simulink model "punto6"  (R2019a)
settings: Solver=VariableStepAuto  StartTime=0.0  StopTime=10.0  MaxStep=1e-4  RelTol=1e-3
values from neighbouring files (symbols this model uses):
  alfa_cu = 3.9 * 10^(-3)    (= 0.0039)    [Datos.m]
  bl = 0    [Datos.m]
  bm = 1.5 * 10^(-5)    (= 1.5e-05)    [Datos.m]
  Cts = 0.818    [Datos.m]
  Id0 = 0.5    [Datos.m]    (also in punto6plot.m)
  Jl = 0.2520    (= 0.252)    [Datos.m]
  Jm = 3.1 * 10^(-6)    (= 3.1e-06)    [Datos.m]
  lambda_m_r = 0.01546    [Datos.m]
  Ld = 6.6e-3    (= 0.0066)    [Datos.m]
  Lq = 5.8e-3    (= 0.0058)    [Datos.m]
  Pp = 3    [Datos.m]
  r = 314.3008    [Datos.m]
  Rts_amb = 146.7    [Datos.m]
  Tlmax = 6.28    [Calculo.m]    (also in Datos.m)
  tstep1 = 0.1    [Calculo.m]    (also in Datos.m)
  tstep2 = 0.3    [Calculo.m]    (also in Datos.m)
  tstep4 = 0.7    [Calculo.m]    (also in Datos.m)
  tstep5 = 0.9    [Calculo.m]    (also in Datos.m)
  Vqsnom = 19.596    [Calculo.m]    (also in Datos.m)
undefined symbols (not defined in the file or in its folder): magnitude
settings Model: Creator=renzo  LastModifiedBy=renzo

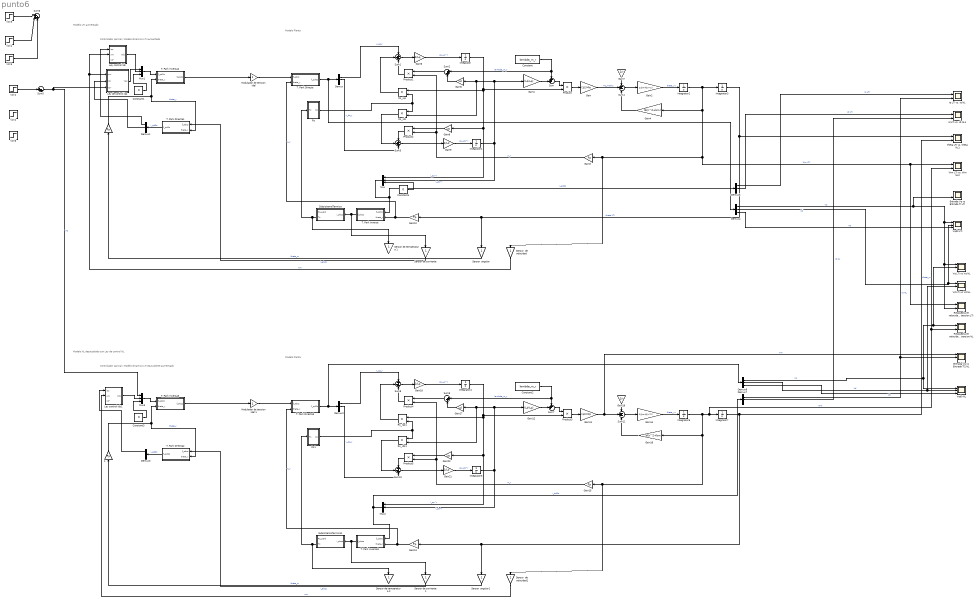
== system punto6 ==
  note: Modelo LTI aumentado
  note: Modelo Planta
  note: Controlador parcial / Modelo dinamico LTI aumentado
  note: Controlador parcial / Modelo dinamico LTI equivalente aumentado
  note: Modelo NL desacoplado con Ley de control NL
  note: Modelo Planta
  " " : Gain  Gain=Pp
  " 1" : Gain  Gain=Pp
  Constant : Constant  Value=lambda_m_r
  Constant1 : Constant  Value=0
  Constant2 : Constant  Value=lambda_m_r
  Constant3 : Constant  Value=0
  Constant4 : Constant  Value=0
  Demux{,1..5,7..8} (8 alike) : Demux  Outputs=3
  Entrada Vq vs Entrada Tl LTI : Scope  NumInputPorts=2
  Entrada Vq vs Entrada Tl2 NL : Scope  NumInputPorts=3
  Gain : Gain  Gain=(3/2)*Pp
  Gain1 : Gain  Gain=(Ld-Lq)
  Gain{3,10,13,15} (4 alike) : Gain  Gain=Pp
  Gain11 : Gain  Gain=(3/2)*Pp
  Gain12 : Gain  Gain=(Ld-Lq)
  Gain14 : Gain  Gain=1/(Jm+Jl/r^2)
  Gain16 : Gain  Gain=bl/r^2+bm
  Gain17 : Gain  Gain=Ld
  Gain18 : Gain  Gain=1/Lq
  Gain19 : Gain  Gain=1/r
  Gain2 : Gain  Gain=1/(Jm+Jl/r^2)
  Gain20 : Gain  Gain=Lq
  Gain21 : Gain  Gain=1/Ld
  Gain4 : Gain  Gain=(bl/r^2+bm)
  Gain5 : Gain  Gain=Ld
  Gain6 : Gain  Gain=1/Lq
  Gain7 : Gain  Gain=1/r
  Gain8 : Gain  Gain=Lq
  Gain9 : Gain  Gain=1/Ld
  Id LTI vs. Id NL1 : Scope  NumInputPorts=2
  Integrator{,2..4,6..7} (6 alike) : Integrator
  Integrator1 : Integrator  InitialCondition=Id0
  Integrator5 : Integrator  InitialCondition=Id0
  Iq LTI vs. Iq NL : Scope  NumInputPorts=2
  Ley control ids : Subsystem
  Ley control ids1 : Subsystem
  Ley de control iqs : Subsystem
  "Modulador de tension idel " : Gain
  Modulador de tension idel 1 : Gain
  Mux{,1..3} (4 alike) : Mux  Inputs=3
  Product{,1..5} (6 alike) : Product
  Respuesta en velocidad vs entrada tension LTI : Scope  NumInputPorts=2
  Respuesta en velocidad vs entrada tension NL : Scope  NumInputPorts=2
  Rs : Subsystem
  Rs1 : Subsystem
  Rs_ids : Product
  Rs_ids1 : Product
  Rs_iqs : Product
  Rs_iqs1 : Product
  Sensor  angular : Gain
  Sensor  angular1 : Gain
  Sensor  de velocidad : Gain
  Sensor  de velocidad1 : Gain
  "Sensor de corriente " : Gain
  Sensor de corriente 1 : Gain
  Sensor de temperatura 1 : Gain
  Sensor de temperatura 2 : Gain
  SubsistemaTermico : Subsystem
  SubsistemaTermico1 : Subsystem
  Sum : Sum  Inputs=++|
  Sum1 : Sum  Inputs=+--
  Sum10 : Sum  Inputs=+-+
  Sum11 : Sum  Inputs=-+-
  Sum2 : Sum  Inputs=|++
  Sum3 : Sum  Inputs=+-+
  Sum4 : Sum  Inputs=-+-
  Sum5 : Sum  Inputs=|++
  Sum6 : Sum  Inputs=|+++
  Sum7 : Sum  Inputs=++|
  Sum8 : Sum  Inputs=+--
  Sum9 : Sum  Inputs=|++
  T. Park Directa : Subsystem
  T. Park Directa1 : Subsystem
  T. Park Directa2 : Subsystem
  T. Park Directa3 : Subsystem
  T. Park Inversa : Subsystem
  T. Park Inversa2 : Subsystem
  T. Park Inversa3 : Subsystem
  T. Park Inversa5 : Subsystem
  V1*1 : Step  Time=tstep1  After=Vqsnom  SampleTime=0
  V1*2 : Step  Time=tstep4  After=-Vqsnom  SampleTime=0
  V1*3 : Step  Time=tstep2  After=Tlmax  SampleTime=0
  V1*4 : Step  Time=tstep4  After=-2*Tlmax  SampleTime=0
  V1*5 : Step  Time=tstep5  After=Tlmax  SampleTime=0
  V1*6 : Step  Time=0.5  After=0  SampleTime=0
  Vd LTI vs Vd NL : Scope  NumInputPorts=3
  Vq LTI vs Vq NL : Scope  NumInputPorts=3
  "Vqd0 LTI " : Scope  NumInputPorts=3
  "Vqd0 NL " : Scope  NumInputPorts=3
  Wm LTI vs. Wm NL2 : Scope  NumInputPorts=2
  theta LTI vs. theta NL1 : Scope  NumInputPorts=2
  wires:
  Gain8/1 -> Product2/1
  Sum1/1 -> Gain6/1
  Product2/1 -> Sum3/1
  Gain5/1 -> Sum2/2
  Demux/1 -> Sum1/1  "v_qs_r"
  Constant/1 -> Sum/1, Sum2/1  "lambda_m_r"
  Gain6/1 -> Integrator/1  "d_i_qr^r"
  Rs_iqs/1 -> Sum1/2
  Product1/1 -> Sum1/3
  Gain9/1 -> Integrator1/1  "d_i_ds^r"
  Integrator/1 -> Product/2, Mux/1, Gain8/1, Rs_iqs/1  "i_qs^r"
  Demux/2 -> Sum3/3  "v_ds_r"
  Gain1/1 -> Sum/2
  Sum2/1 -> Product1/1
  Sum3/1 -> Gain9/1
  Gain3/1 -> Product1/2, Product2/2  "w_r"
  Sum/1 -> Product/1
  Rs_ids/1 -> Sum3/2
  Integrator1/1 -> Gain5/1, Rs_ids/2, Gain1/1, Mux/2  "i_ds^r"
  Mux/1 -> T. Park Inversa/1(f_qd0s), Demux5/1  "i_qd0s"
  Product/1 -> Gain/1
  Gain2/1 -> Integrator2/1  "theta_vv"
  Gain4/1 -> Sum4/3
  Gain/1 -> Sum4/2  "Tq_motriz"
  Sum4/1 -> Gain2/1
  Rs/1(Rs) -> Rs_ids/1, Rs_iqs/2
  SubsistemaTermico/2(Ts) -> Sensor de temperatura 1/1, Rs/1(Ts)
  Gain7/1 -> Sum4/1
  T. Park Inversa/1(f_abcs) -> "Sensor de corriente "/1, SubsistemaTermico/1(i_abcs)
  " "/1 -> T. Park Inversa2/2(theta_r), T. Park Directa1/2(theta_r)  "theta_r"
  T. Park Directa1/1(f_qd0s) -> Demux1/1  "i_qd0s"
  Constant1/1 -> Mux1/3
  Ley control ids/1(Vds) -> Mux1/2
  Ley de control iqs/1(Vqs) -> Mux1/1
  Demux1/2 -> Ley de control iqs/2(ids)
  Demux1/1 -> Ley control ids/1(iqs)
  Mux1/1 -> T. Park Inversa2/1(f_qd0s)
  Gain10/1 -> T. Park Directa/2(theta_r), T. Park Inversa/2(theta_r)  "w_r"
  "Modulador de tension idel "/1 -> T. Park Directa/1(f_abcs)
  T. Park Inversa2/1(f_abcs) -> "Modulador de tension idel "/1
  "Sensor de corriente "/1 -> T. Park Directa1/1(f_abcs)  "i_abcs"
  Sensor  angular/1 -> " "/1  "theta_m"
  Sensor  de velocidad/1 -> Ley control ids/2(wm), Ley de control iqs/1(wm)  "wm"
  V1*1/1 -> Sum5/1
  V1*3/1 -> Sum6/1
  V1*5/1 -> Sum6/3
  V1*4/1 -> Sum6/2
  Sum5/1 -> Mux3/1, Ley de control iqs/3(Vq*)  "Vq"
  Mux3/1 -> T. Park Inversa5/1(f_qd0s)
  Ley control ids1/1(Vds) -> Mux3/2
  Constant3/1 -> Mux3/3
  T. Park Directa2/1(f_qd0s) -> Demux3/1  "i_qd0s"
  " 1"/1 -> T. Park Inversa5/2(theta_r), T. Park Directa2/2(theta_r)  "theta_r"
  Sensor  angular1/1 -> " 1"/1  "theta_m"
  T. Park Inversa3/1(f_abcs) -> Sensor de corriente 1/1, SubsistemaTermico1/1(i_abcs)
  Gain14/1 -> Integrator6/1  "theta_vv"
  Rs1/1(Rs) -> Rs_ids1/1, Rs_iqs1/2
  Product3/1 -> Gain11/1
  Rs_ids1/1 -> Sum10/2
  Gain15/1 -> Product4/2, Product5/2  "w_r"
  Sum7/1 -> Product3/1
  Gain16/1 -> Sum11/3
  Gain19/1 -> Sum11/1
  Sum10/1 -> Gain21/1
  Sum9/1 -> Product4/1
  Demux2/2 -> Sum10/3  "v_ds_r"
  Gain21/1 -> Integrator5/1  "d_i_ds^r"
  Rs_iqs1/1 -> Sum8/2
  Product4/1 -> Sum8/3
  Gain18/1 -> Integrator4/1  "d_i_qr^r"
  Constant2/1 -> Sum7/1, Sum9/1  "lambda_m_r"
  Sum8/1 -> Gain18/1
  Product5/1 -> Sum10/1
  Gain17/1 -> Sum9/2
  Integrator4/1 -> Product3/2, Mux2/1, Gain20/1, Rs_iqs1/1  "i_qs^r"
  Gain20/1 -> Product5/1
  Demux2/1 -> Sum8/1  "v_qs_r"
  Modulador de tension idel 1/1 -> T. Park Directa3/1(f_abcs)
  Sum11/1 -> Gain14/1
  SubsistemaTermico1/2(Ts) -> Sensor de temperatura 2/1, Rs1/1(Ts)
  T. Park Directa3/1(f_qd0s) -> Demux8/1, Demux2/1
  Sensor de corriente 1/1 -> T. Park Directa2/1(f_abcs)  "i_abcs"
  Mux2/1 -> T. Park Inversa3/1(f_qd0s), Demux7/1  "i_qd0s"
  Gain12/1 -> Sum7/2
  Gain13/1 -> T. Park Directa3/2(theta_r), T. Park Inversa3/2(theta_r)  "w_r"
  Sensor  de velocidad1/1 -> Ley control ids1/2(wm)  "wm"
  Integrator5/1 -> Gain17/1, Rs_ids1/2, Gain12/1, Mux2/2  "i_ds^r"
  T. Park Inversa5/1(f_abcs) -> Modulador de tension idel 1/1
  Demux7/1 -> Iq LTI vs. Iq NL/2, Entrada Vq vs Entrada Tl2 NL/2  "Iq NL"
  Gain11/1 -> Entrada Vq vs Entrada Tl2 NL/1, Sum11/2  "Tm"
  Demux5/2 -> Id LTI vs. Id NL1/1  "Id LTI"
  Integrator3/1 -> theta LTI vs. theta NL1/1, Sensor  angular/1, Gain10/1  "theta LTI"
  Integrator6/1 -> Sensor  de velocidad1/1, Gain15/1, Gain16/1, Respuesta en velocidad vs entrada tension NL/2, Wm LTI vs. Wm NL2/2, Integrator7/1  "Wm"
  Demux7/2 -> Id LTI vs. Id NL1/2  "Id NL"
  Integrator2/1 -> Respuesta en velocidad vs entrada tension LTI/1, Wm LTI vs. Wm NL2/1, Sensor  de velocidad/1, Gain3/1, Gain4/1, Integrator3/1  "Wm LTI"
  Demux4/2 -> "Vqd0 LTI "/2, Vd LTI vs Vd NL/1  "Vd"
  Integrator7/1 -> theta LTI vs. theta NL1/2, Sensor  angular1/1, Gain13/1  "theta_m"
  Demux4/1 -> Respuesta en velocidad vs entrada tension LTI/2, Vq LTI vs Vq NL/1, "Vqd0 LTI "/1, Entrada Vq vs Entrada Tl LTI/2  "Vq"
  Demux4/3 -> "Vqd0 LTI "/3  "V0"
  Demux5/1 -> Iq LTI vs. Iq NL/1  "Iq LTI"
  T. Park Directa/1(f_qd0s) -> Demux4/1, Demux/1
  Demux8/1 -> Respuesta en velocidad vs entrada tension NL/1, Vq LTI vs Vq NL/2, "Vqd0 NL "/1  "Vq"
  Demux8/2 -> "Vqd0 NL "/2, Vd LTI vs Vd NL/2  "Vd"
  Demux8/3 -> "Vqd0 NL "/3  "V0"
  Demux3/1 -> Ley control ids1/1(iqs)
  Constant4/1 -> Mux/3

== system punto6/Ley control ids ==
  iqs : Inport
  wm : Inport  Port=2
  Vd* : Inport  Port=3
  Ley de Control minima : Subsystem
  Sum : Sum  Inputs=|-+
  Vds : Outport
  wires:
  wm/1 -> Ley de Control minima/2(wm)
  iqs/1 -> Ley de Control minima/1(Iqs)
  Ley de Control minima/1(Vds*) -> Sum/1
  Sum/1 -> Vds/1
  Vd*/1 -> Sum/2

== system punto6/Ley control ids1 ==
  iqs : Inport
  wm : Inport  Port=2
  Vd* : Inport  Port=3
  Ley de Control minima : Subsystem
  Sum : Sum  Inputs=|-+
  Vds : Outport
  wires:
  wm/1 -> Ley de Control minima/2(wm)
  iqs/1 -> Ley de Control minima/1(Iqs)
  Ley de Control minima/1(Vds*) -> Sum/1
  Sum/1 -> Vds/1
  Vd*/1 -> Sum/2

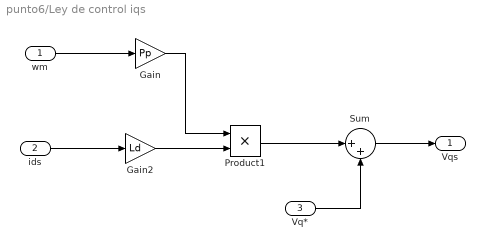
== system punto6/Ley de control iqs ==
  wm : Inport
  ids : Inport  Port=2
  Vq* : Inport  Port=3
  Gain : Gain  Gain=Pp
  Gain2 : Gain  Gain=Ld
  Product1 : Product
  Sum : Sum  Inputs=|++
  Vqs : Outport
  wires:
  wm/1 -> Gain/1
  Gain/1 -> Product1/1
  ids/1 -> Gain2/1
  Gain2/1 -> Product1/2
  Product1/1 -> Sum/1
  Sum/1 -> Vqs/1
  Vq*/1 -> Sum/2

== system punto6/Rs ==
  Ts : Inport
  Rs_ref : Gain  Gain=1.02
  Sum5 : Sum  Inputs=|+-
  Sum6 : Sum  Inputs=|++
  Ts_ref : Constant  Value=40
  alfa_cu : Gain  Gain=alfa_cu
  cte : Constant
  Rs : Outport
  wires:
  Ts_ref/1 -> Sum5/2
  Sum5/1 -> alfa_cu/1
  Sum6/1 -> Rs_ref/1
  Ts/1 -> Sum5/1
  alfa_cu/1 -> Sum6/1
  cte/1 -> Sum6/2
  Rs_ref/1 -> Rs/1  "Rs"

== system punto6/Rs1 ==
  Ts : Inport
  Rs_ref : Gain  Gain=1.02
  Sum5 : Sum  Inputs=|+-
  Sum6 : Sum  Inputs=|++
  Ts_ref : Constant  Value=40
  alfa_cu : Gain  Gain=alfa_cu
  cte : Constant
  Rs : Outport
  wires:
  Ts_ref/1 -> Sum5/2
  Sum5/1 -> alfa_cu/1
  Sum6/1 -> Rs_ref/1
  Ts/1 -> Sum5/1
  alfa_cu/1 -> Sum6/1
  cte/1 -> Sum6/2
  Rs_ref/1 -> Rs/1  "Rs"

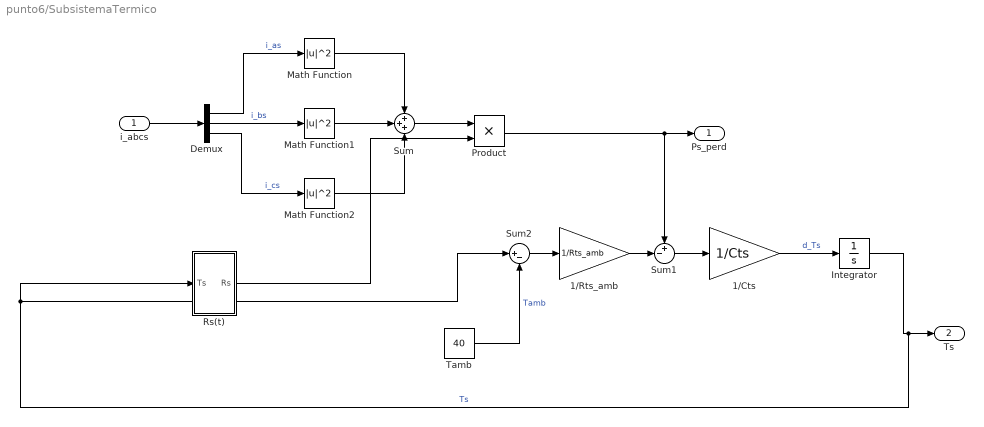
== system punto6/SubsistemaTermico ==
  i_abcs : Inport
  1/Cts : Gain  Gain=1/Cts
  1/Rts_amb : Gain  Gain=1/Rts_amb
  Demux : Demux  Outputs=3
  Integrator : Integrator  InitialCondition=40
  Math Function : Math  Operator=magnitude^2  SaturateOnIntegerOverflow=on
  Math Function1 : Math  Operator=magnitude^2  SaturateOnIntegerOverflow=on
  Math Function2 : Math  Operator=magnitude^2  SaturateOnIntegerOverflow=on
  Product : Product
  Rs(t) : Subsystem
  Sum : Sum  Inputs=3
  Sum1 : Sum  Inputs=+-|
  Sum2 : Sum  Inputs=|+-
  Tamb : Constant  Value=40
  Ps_perd : Outport  VectorParamsAs1DForOutWhenUnconnected=on
  Ts : Outport  Port=2  VectorParamsAs1DForOutWhenUnconnected=on
  wires:
  i_abcs/1 -> Demux/1
  Demux/1 -> Math Function/1  "i_as"
  Demux/2 -> Math Function1/1  "i_bs"
  Demux/3 -> Math Function2/1  "i_cs"
  Math Function1/1 -> Sum/2
  Math Function/1 -> Sum/1
  Math Function2/1 -> Sum/3
  Sum/1 -> Product/1
  Product/1 -> Sum1/1, Ps_perd/1
  Tamb/1 -> Sum2/2  "Tamb"
  Sum2/1 -> 1/Rts_amb/1
  1/Rts_amb/1 -> Sum1/2
  Sum1/1 -> 1/Cts/1
  1/Cts/1 -> Integrator/1  "d_Ts"
  Integrator/1 -> Rs(t)/1(Ts), Sum2/1, Ts/1  "Ts"
  Rs(t)/1(Rs) -> Product/2

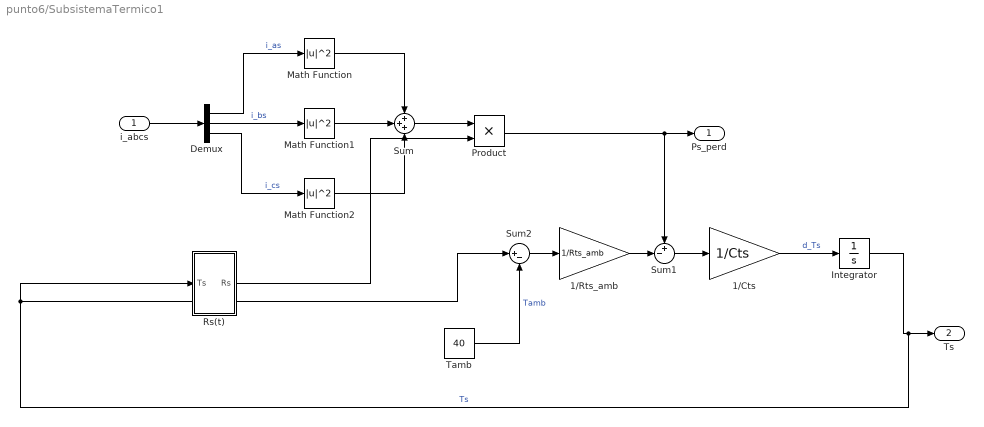
== system punto6/SubsistemaTermico1 ==
  i_abcs : Inport
  1/Cts : Gain  Gain=1/Cts
  1/Rts_amb : Gain  Gain=1/Rts_amb
  Demux : Demux  Outputs=3
  Integrator : Integrator  InitialCondition=40
  Math Function : Math  Operator=magnitude^2  SaturateOnIntegerOverflow=on
  Math Function1 : Math  Operator=magnitude^2  SaturateOnIntegerOverflow=on
  Math Function2 : Math  Operator=magnitude^2  SaturateOnIntegerOverflow=on
  Product : Product
  Rs(t) : Subsystem
  Sum : Sum  Inputs=3
  Sum1 : Sum  Inputs=+-|
  Sum2 : Sum  Inputs=|+-
  Tamb : Constant  Value=40
  Ps_perd : Outport  VectorParamsAs1DForOutWhenUnconnected=on
  Ts : Outport  Port=2  VectorParamsAs1DForOutWhenUnconnected=on
  wires:
  i_abcs/1 -> Demux/1
  Demux/1 -> Math Function/1  "i_as"
  Demux/2 -> Math Function1/1  "i_bs"
  Demux/3 -> Math Function2/1  "i_cs"
  Math Function1/1 -> Sum/2
  Math Function/1 -> Sum/1
  Math Function2/1 -> Sum/3
  Sum/1 -> Product/1
  Product/1 -> Sum1/1, Ps_perd/1
  Tamb/1 -> Sum2/2  "Tamb"
  Sum2/1 -> 1/Rts_amb/1
  1/Rts_amb/1 -> Sum1/2
  Sum1/1 -> 1/Cts/1
  1/Cts/1 -> Integrator/1  "d_Ts"
  Integrator/1 -> Rs(t)/1(Ts), Sum2/1, Ts/1  "Ts"
  Rs(t)/1(Rs) -> Product/2

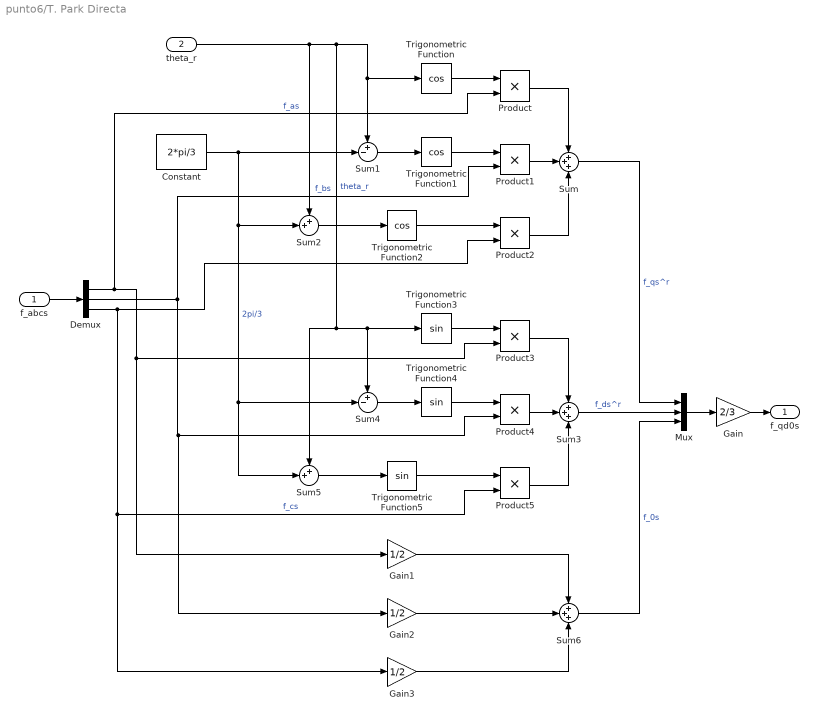
== system punto6/T. Park Directa ==
  f_abcs : Inport
  theta_r : Inport  Port=2
  Constant : Constant  Value=2*pi/3
  Demux : Demux  Outputs=3
  Gain : Gain  Gain=2/3
  Gain1 : Gain  Gain=1/2
  Gain2 : Gain  Gain=1/2
  Gain3 : Gain  Gain=1/2
  Mux : Mux  Inputs=3
  Product{,1..5} (6 alike) : Product
  Sum : Sum  Inputs=3
  Sum1 : Sum  Inputs=+-|
  Sum2 : Sum  Inputs=++|
  Sum3 : Sum  Inputs=3
  Sum4 : Sum  Inputs=+-|
  Sum5 : Sum  Inputs=++|
  Sum6 : Sum  Inputs=3
  Trigonometric Function : Trigonometry  Operator=cos
  Trigonometric Function1 : Trigonometry  Operator=cos
  Trigonometric Function2 : Trigonometry  Operator=cos
  Trigonometric Function3 : Trigonometry
  Trigonometric Function4 : Trigonometry
  Trigonometric Function5 : Trigonometry
  f_qd0s : Outport  VectorParamsAs1DForOutWhenUnconnected=on
  wires:
  Mux/1 -> Gain/1
  f_abcs/1 -> Demux/1
  Demux/1 -> Gain1/1, Product3/2, Product/2  "f_as"
  Demux/2 -> Gain2/1, Product4/2, Product1/2  "f_bs"
  Demux/3 -> Gain3/1, Product5/2, Product2/2  "f_cs"
  Sum/1 -> Mux/1  "f_qs^r"
  Gain/1 -> f_qd0s/1
  Trigonometric Function/1 -> Product/1
  Product/1 -> Sum/1
  Sum1/1 -> Trigonometric Function1/1
  Constant/1 -> Sum5/2, Sum4/2, Sum2/2, Sum1/2  "2pi/3"
  Trigonometric Function1/1 -> Product1/1
  Product1/1 -> Sum/2
  Product2/1 -> Sum/3
  Trigonometric Function2/1 -> Product2/1
  Sum2/1 -> Trigonometric Function2/1
  Product4/1 -> Sum3/2
  Trigonometric Function5/1 -> Product5/1
  Sum5/1 -> Trigonometric Function5/1
  Product5/1 -> Sum3/3
  Product3/1 -> Sum3/1
  Trigonometric Function4/1 -> Product4/1
  Sum4/1 -> Trigonometric Function4/1
  Sum3/1 -> Mux/2  "f_ds^r"
  Trigonometric Function3/1 -> Product3/1
  theta_r/1 -> Sum5/1, Sum4/1, Trigonometric Function3/1, Trigonometric Function/1, Sum1/1, Sum2/1  "theta_r"
  Sum6/1 -> Mux/3  "f_0s"
  Gain3/1 -> Sum6/3
  Gain1/1 -> Sum6/1
  Gain2/1 -> Sum6/2

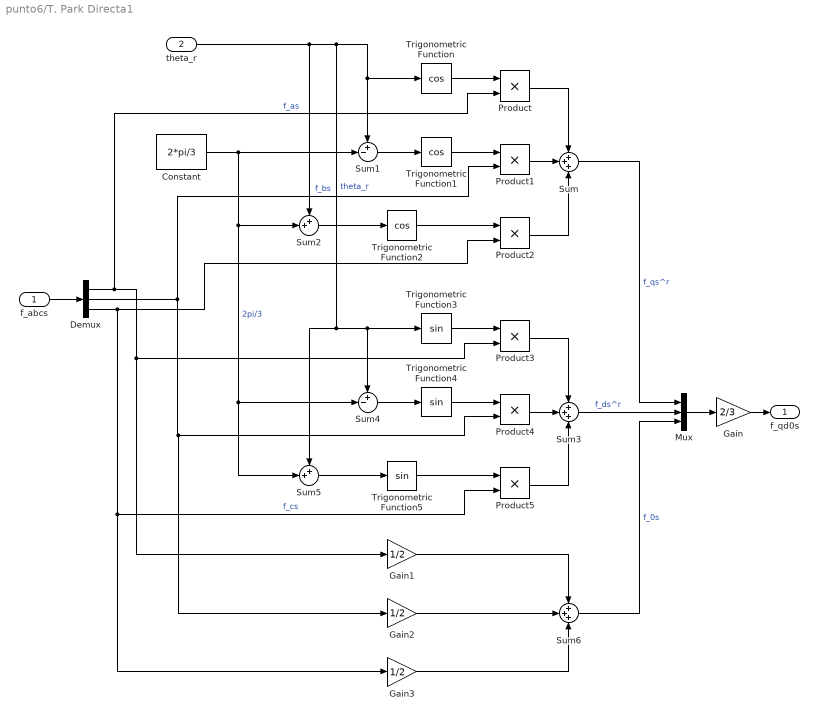
== system punto6/T. Park Directa1 ==
  f_abcs : Inport
  theta_r : Inport  Port=2
  Constant : Constant  Value=2*pi/3
  Demux : Demux  Outputs=3
  Gain : Gain  Gain=2/3
  Gain1 : Gain  Gain=1/2
  Gain2 : Gain  Gain=1/2
  Gain3 : Gain  Gain=1/2
  Mux : Mux  Inputs=3
  Product{,1..5} (6 alike) : Product
  Sum : Sum  Inputs=3
  Sum1 : Sum  Inputs=+-|
  Sum2 : Sum  Inputs=++|
  Sum3 : Sum  Inputs=3
  Sum4 : Sum  Inputs=+-|
  Sum5 : Sum  Inputs=++|
  Sum6 : Sum  Inputs=3
  Trigonometric Function : Trigonometry  Operator=cos
  Trigonometric Function1 : Trigonometry  Operator=cos
  Trigonometric Function2 : Trigonometry  Operator=cos
  Trigonometric Function3 : Trigonometry
  Trigonometric Function4 : Trigonometry
  Trigonometric Function5 : Trigonometry
  f_qd0s : Outport  VectorParamsAs1DForOutWhenUnconnected=on
  wires:
  Mux/1 -> Gain/1
  f_abcs/1 -> Demux/1
  Demux/1 -> Gain1/1, Product3/2, Product/2  "f_as"
  Demux/2 -> Gain2/1, Product4/2, Product1/2  "f_bs"
  Demux/3 -> Gain3/1, Product5/2, Product2/2  "f_cs"
  Sum/1 -> Mux/1  "f_qs^r"
  Gain/1 -> f_qd0s/1
  Trigonometric Function/1 -> Product/1
  Product/1 -> Sum/1
  Sum1/1 -> Trigonometric Function1/1
  Constant/1 -> Sum5/2, Sum4/2, Sum2/2, Sum1/2  "2pi/3"
  Trigonometric Function1/1 -> Product1/1
  Product1/1 -> Sum/2
  Product2/1 -> Sum/3
  Trigonometric Function2/1 -> Product2/1
  Sum2/1 -> Trigonometric Function2/1
  Product4/1 -> Sum3/2
  Trigonometric Function5/1 -> Product5/1
  Sum5/1 -> Trigonometric Function5/1
  Product5/1 -> Sum3/3
  Product3/1 -> Sum3/1
  Trigonometric Function4/1 -> Product4/1
  Sum4/1 -> Trigonometric Function4/1
  Sum3/1 -> Mux/2  "f_ds^r"
  Trigonometric Function3/1 -> Product3/1
  theta_r/1 -> Sum5/1, Sum4/1, Trigonometric Function3/1, Trigonometric Function/1, Sum1/1, Sum2/1  "theta_r"
  Sum6/1 -> Mux/3  "f_0s"
  Gain3/1 -> Sum6/3
  Gain1/1 -> Sum6/1
  Gain2/1 -> Sum6/2

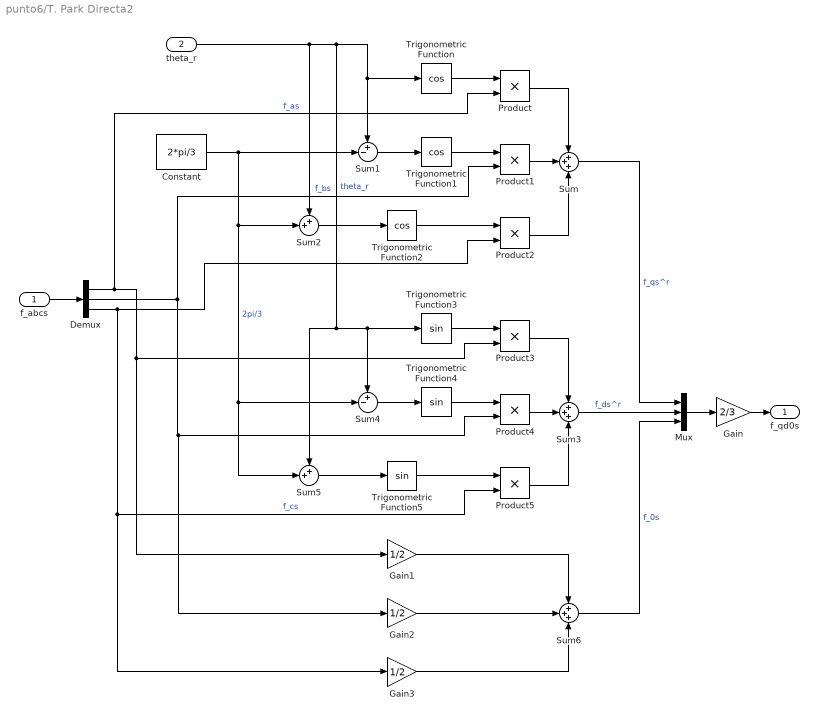
== system punto6/T. Park Directa2 ==
  f_abcs : Inport
  theta_r : Inport  Port=2
  Constant : Constant  Value=2*pi/3
  Demux : Demux  Outputs=3
  Gain : Gain  Gain=2/3
  Gain1 : Gain  Gain=1/2
  Gain2 : Gain  Gain=1/2
  Gain3 : Gain  Gain=1/2
  Mux : Mux  Inputs=3
  Product{,1..5} (6 alike) : Product
  Sum : Sum  Inputs=3
  Sum1 : Sum  Inputs=+-|
  Sum2 : Sum  Inputs=++|
  Sum3 : Sum  Inputs=3
  Sum4 : Sum  Inputs=+-|
  Sum5 : Sum  Inputs=++|
  Sum6 : Sum  Inputs=3
  Trigonometric Function : Trigonometry  Operator=cos
  Trigonometric Function1 : Trigonometry  Operator=cos
  Trigonometric Function2 : Trigonometry  Operator=cos
  Trigonometric Function3 : Trigonometry
  Trigonometric Function4 : Trigonometry
  Trigonometric Function5 : Trigonometry
  f_qd0s : Outport  VectorParamsAs1DForOutWhenUnconnected=on
  wires:
  Mux/1 -> Gain/1
  f_abcs/1 -> Demux/1
  Demux/1 -> Gain1/1, Product3/2, Product/2  "f_as"
  Demux/2 -> Gain2/1, Product4/2, Product1/2  "f_bs"
  Demux/3 -> Gain3/1, Product5/2, Product2/2  "f_cs"
  Sum/1 -> Mux/1  "f_qs^r"
  Gain/1 -> f_qd0s/1
  Trigonometric Function/1 -> Product/1
  Product/1 -> Sum/1
  Sum1/1 -> Trigonometric Function1/1
  Constant/1 -> Sum5/2, Sum4/2, Sum2/2, Sum1/2  "2pi/3"
  Trigonometric Function1/1 -> Product1/1
  Product1/1 -> Sum/2
  Product2/1 -> Sum/3
  Trigonometric Function2/1 -> Product2/1
  Sum2/1 -> Trigonometric Function2/1
  Product4/1 -> Sum3/2
  Trigonometric Function5/1 -> Product5/1
  Sum5/1 -> Trigonometric Function5/1
  Product5/1 -> Sum3/3
  Product3/1 -> Sum3/1
  Trigonometric Function4/1 -> Product4/1
  Sum4/1 -> Trigonometric Function4/1
  Sum3/1 -> Mux/2  "f_ds^r"
  Trigonometric Function3/1 -> Product3/1
  theta_r/1 -> Sum5/1, Sum4/1, Trigonometric Function3/1, Trigonometric Function/1, Sum1/1, Sum2/1  "theta_r"
  Sum6/1 -> Mux/3  "f_0s"
  Gain3/1 -> Sum6/3
  Gain1/1 -> Sum6/1
  Gain2/1 -> Sum6/2

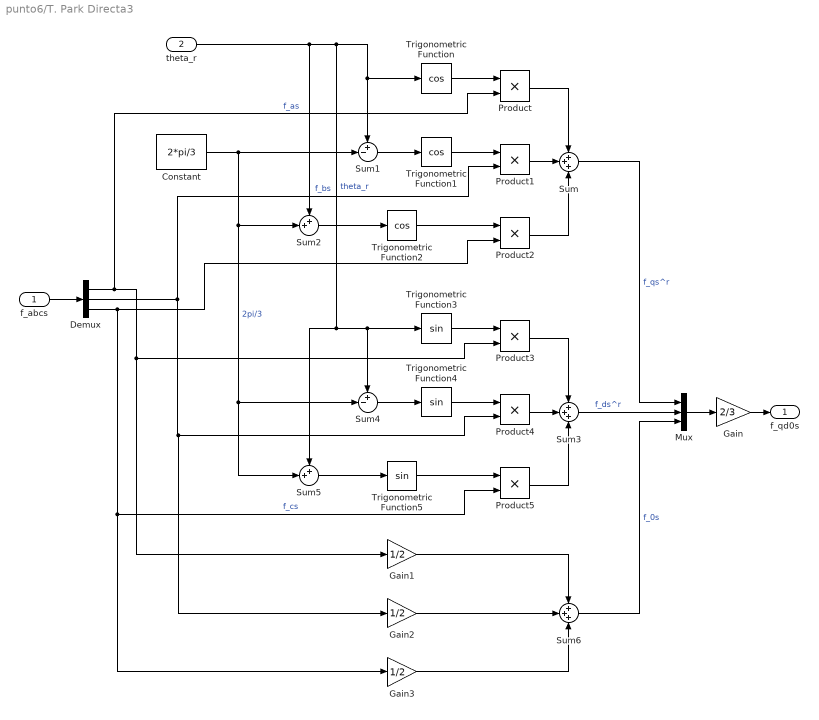
== system punto6/T. Park Directa3 ==
  f_abcs : Inport
  theta_r : Inport  Port=2
  Constant : Constant  Value=2*pi/3
  Demux : Demux  Outputs=3
  Gain : Gain  Gain=2/3
  Gain1 : Gain  Gain=1/2
  Gain2 : Gain  Gain=1/2
  Gain3 : Gain  Gain=1/2
  Mux : Mux  Inputs=3
  Product{,1..5} (6 alike) : Product
  Sum : Sum  Inputs=3
  Sum1 : Sum  Inputs=+-|
  Sum2 : Sum  Inputs=++|
  Sum3 : Sum  Inputs=3
  Sum4 : Sum  Inputs=+-|
  Sum5 : Sum  Inputs=++|
  Sum6 : Sum  Inputs=3
  Trigonometric Function : Trigonometry  Operator=cos
  Trigonometric Function1 : Trigonometry  Operator=cos
  Trigonometric Function2 : Trigonometry  Operator=cos
  Trigonometric Function3 : Trigonometry
  Trigonometric Function4 : Trigonometry
  Trigonometric Function5 : Trigonometry
  f_qd0s : Outport  VectorParamsAs1DForOutWhenUnconnected=on
  wires:
  Mux/1 -> Gain/1
  f_abcs/1 -> Demux/1
  Demux/1 -> Gain1/1, Product3/2, Product/2  "f_as"
  Demux/2 -> Gain2/1, Product4/2, Product1/2  "f_bs"
  Demux/3 -> Gain3/1, Product5/2, Product2/2  "f_cs"
  Sum/1 -> Mux/1  "f_qs^r"
  Gain/1 -> f_qd0s/1
  Trigonometric Function/1 -> Product/1
  Product/1 -> Sum/1
  Sum1/1 -> Trigonometric Function1/1
  Constant/1 -> Sum5/2, Sum4/2, Sum2/2, Sum1/2  "2pi/3"
  Trigonometric Function1/1 -> Product1/1
  Product1/1 -> Sum/2
  Product2/1 -> Sum/3
  Trigonometric Function2/1 -> Product2/1
  Sum2/1 -> Trigonometric Function2/1
  Product4/1 -> Sum3/2
  Trigonometric Function5/1 -> Product5/1
  Sum5/1 -> Trigonometric Function5/1
  Product5/1 -> Sum3/3
  Product3/1 -> Sum3/1
  Trigonometric Function4/1 -> Product4/1
  Sum4/1 -> Trigonometric Function4/1
  Sum3/1 -> Mux/2  "f_ds^r"
  Trigonometric Function3/1 -> Product3/1
  theta_r/1 -> Sum5/1, Sum4/1, Trigonometric Function3/1, Trigonometric Function/1, Sum1/1, Sum2/1  "theta_r"
  Sum6/1 -> Mux/3  "f_0s"
  Gain3/1 -> Sum6/3
  Gain1/1 -> Sum6/1
  Gain2/1 -> Sum6/2

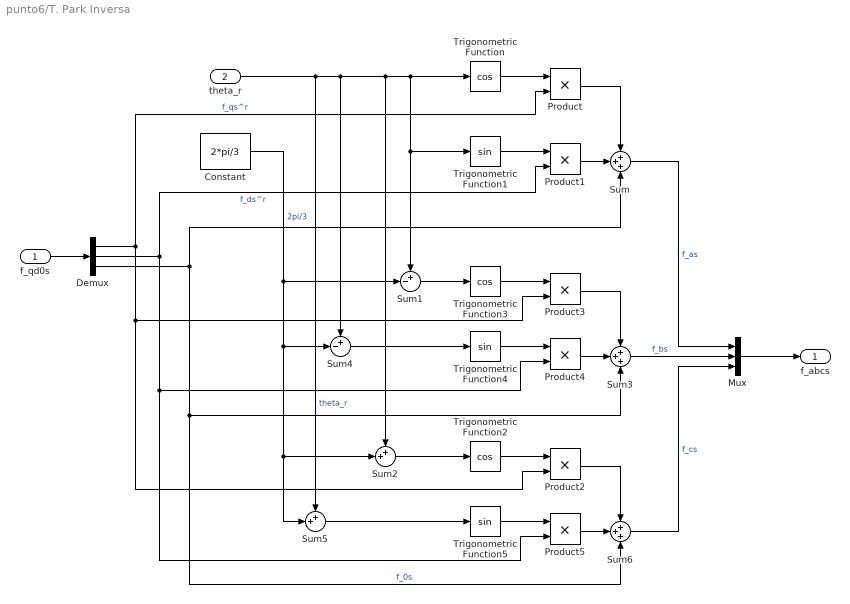
== system punto6/T. Park Inversa ==
  f_qd0s : Inport
  theta_r : Inport  Port=2
  Constant : Constant  Value=2*pi/3
  Demux : Demux  Outputs=3
  Mux : Mux  Inputs=3
  Product{,1..5} (6 alike) : Product
  Sum : Sum  Inputs=3
  Sum1 : Sum  Inputs=+-|
  Sum2 : Sum  Inputs=++|
  Sum3 : Sum  Inputs=3
  Sum4 : Sum  Inputs=+-|
  Sum5 : Sum  Inputs=++|
  Sum6 : Sum  Inputs=3
  Trigonometric Function : Trigonometry  Operator=cos
  Trigonometric Function1 : Trigonometry
  Trigonometric Function2 : Trigonometry  Operator=cos
  Trigonometric Function3 : Trigonometry  Operator=cos
  Trigonometric Function4 : Trigonometry
  Trigonometric Function5 : Trigonometry
  f_abcs : Outport  VectorParamsAs1DForOutWhenUnconnected=on
  wires:
  Trigonometric Function4/1 -> Product4/1
  f_qd0s/1 -> Demux/1
  Trigonometric Function/1 -> Product/1
  Constant/1 -> Sum1/2, Sum4/2, Sum2/2, Sum5/2  "2pi/3"
  Product1/1 -> Sum/2
  Mux/1 -> f_abcs/1
  Sum6/1 -> Mux/3  "f_cs"
  Product/1 -> Sum/1
  theta_r/1 -> Trigonometric Function/1, Trigonometric Function1/1, Sum1/1, Sum2/1, Sum4/1, Sum5/1  "theta_r"
  Product4/1 -> Sum3/2
  Sum3/1 -> Mux/2  "f_bs"
  Trigonometric Function1/1 -> Product1/1
  Sum/1 -> Mux/1  "f_as"
  Trigonometric Function3/1 -> Product3/1
  Product3/1 -> Sum3/1
  Sum4/1 -> Trigonometric Function4/1
  Demux/1 -> Product2/2, Product3/2, Product/2  "f_qs^r"
  Demux/2 -> Product5/2, Product4/2, Product1/2  "f_ds^r"
  Demux/3 -> Sum/3, Sum6/3, Sum3/3  "f_0s"
  Sum1/1 -> Trigonometric Function3/1
  Sum5/1 -> Trigonometric Function5/1
  Trigonometric Function5/1 -> Product5/1
  Trigonometric Function2/1 -> Product2/1
  Product2/1 -> Sum6/1
  Product5/1 -> Sum6/2
  Sum2/1 -> Trigonometric Function2/1

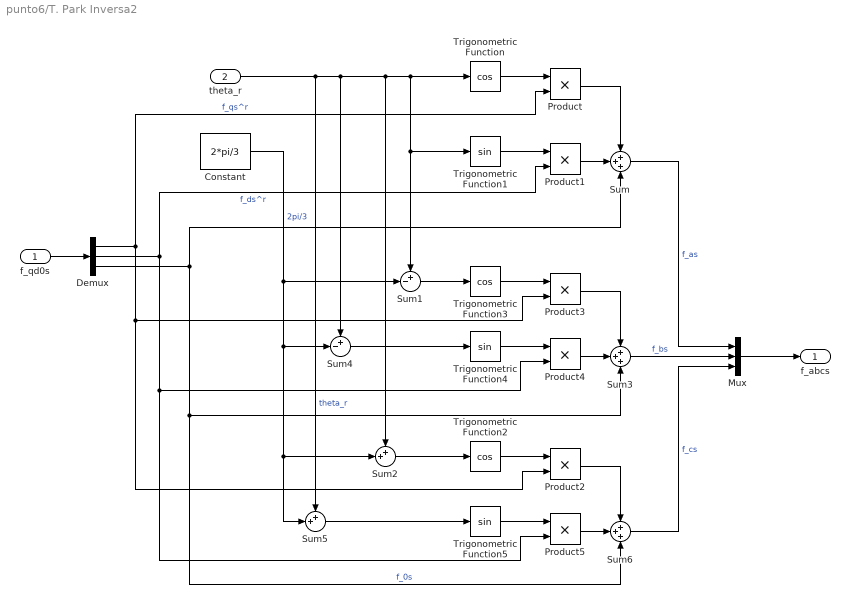
== system punto6/T. Park Inversa2 ==
  f_qd0s : Inport
  theta_r : Inport  Port=2
  Constant : Constant  Value=2*pi/3
  Demux : Demux  Outputs=3
  Mux : Mux  Inputs=3
  Product{,1..5} (6 alike) : Product
  Sum : Sum  Inputs=3
  Sum1 : Sum  Inputs=+-|
  Sum2 : Sum  Inputs=++|
  Sum3 : Sum  Inputs=3
  Sum4 : Sum  Inputs=+-|
  Sum5 : Sum  Inputs=++|
  Sum6 : Sum  Inputs=3
  Trigonometric Function : Trigonometry  Operator=cos
  Trigonometric Function1 : Trigonometry
  Trigonometric Function2 : Trigonometry  Operator=cos
  Trigonometric Function3 : Trigonometry  Operator=cos
  Trigonometric Function4 : Trigonometry
  Trigonometric Function5 : Trigonometry
  f_abcs : Outport  VectorParamsAs1DForOutWhenUnconnected=on
  wires:
  Trigonometric Function4/1 -> Product4/1
  f_qd0s/1 -> Demux/1
  Trigonometric Function/1 -> Product/1
  Constant/1 -> Sum1/2, Sum4/2, Sum2/2, Sum5/2  "2pi/3"
  Product1/1 -> Sum/2
  Mux/1 -> f_abcs/1
  Sum6/1 -> Mux/3  "f_cs"
  Product/1 -> Sum/1
  theta_r/1 -> Trigonometric Function/1, Trigonometric Function1/1, Sum1/1, Sum2/1, Sum4/1, Sum5/1  "theta_r"
  Product4/1 -> Sum3/2
  Sum3/1 -> Mux/2  "f_bs"
  Trigonometric Function1/1 -> Product1/1
  Sum/1 -> Mux/1  "f_as"
  Trigonometric Function3/1 -> Product3/1
  Product3/1 -> Sum3/1
  Sum4/1 -> Trigonometric Function4/1
  Demux/1 -> Product2/2, Product3/2, Product/2  "f_qs^r"
  Demux/2 -> Product5/2, Product4/2, Product1/2  "f_ds^r"
  Demux/3 -> Sum/3, Sum6/3, Sum3/3  "f_0s"
  Sum1/1 -> Trigonometric Function3/1
  Sum5/1 -> Trigonometric Function5/1
  Trigonometric Function5/1 -> Product5/1
  Trigonometric Function2/1 -> Product2/1
  Product2/1 -> Sum6/1
  Product5/1 -> Sum6/2
  Sum2/1 -> Trigonometric Function2/1

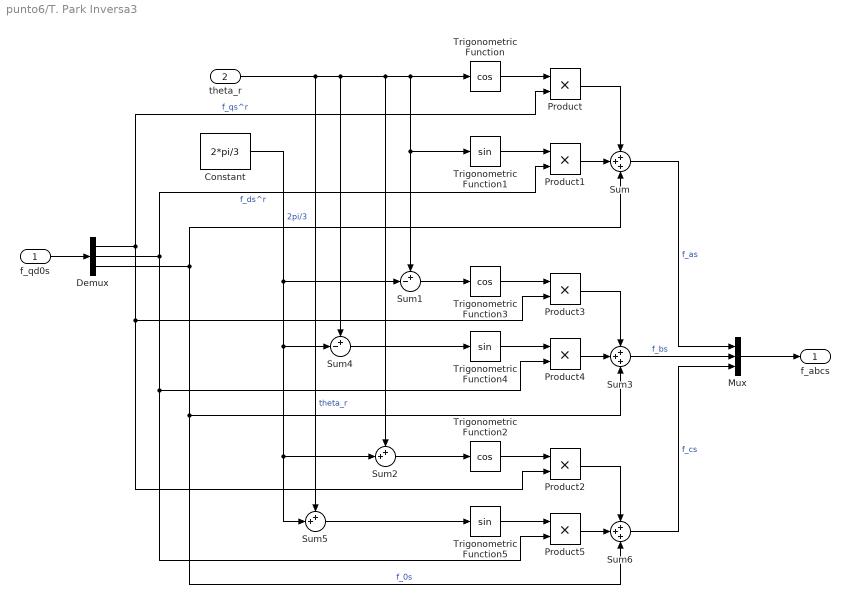
== system punto6/T. Park Inversa3 ==
  f_qd0s : Inport
  theta_r : Inport  Port=2
  Constant : Constant  Value=2*pi/3
  Demux : Demux  Outputs=3
  Mux : Mux  Inputs=3
  Product{,1..5} (6 alike) : Product
  Sum : Sum  Inputs=3
  Sum1 : Sum  Inputs=+-|
  Sum2 : Sum  Inputs=++|
  Sum3 : Sum  Inputs=3
  Sum4 : Sum  Inputs=+-|
  Sum5 : Sum  Inputs=++|
  Sum6 : Sum  Inputs=3
  Trigonometric Function : Trigonometry  Operator=cos
  Trigonometric Function1 : Trigonometry
  Trigonometric Function2 : Trigonometry  Operator=cos
  Trigonometric Function3 : Trigonometry  Operator=cos
  Trigonometric Function4 : Trigonometry
  Trigonometric Function5 : Trigonometry
  f_abcs : Outport  VectorParamsAs1DForOutWhenUnconnected=on
  wires:
  Trigonometric Function4/1 -> Product4/1
  f_qd0s/1 -> Demux/1
  Trigonometric Function/1 -> Product/1
  Constant/1 -> Sum1/2, Sum4/2, Sum2/2, Sum5/2  "2pi/3"
  Product1/1 -> Sum/2
  Mux/1 -> f_abcs/1
  Sum6/1 -> Mux/3  "f_cs"
  Product/1 -> Sum/1
  theta_r/1 -> Trigonometric Function/1, Trigonometric Function1/1, Sum1/1, Sum2/1, Sum4/1, Sum5/1  "theta_r"
  Product4/1 -> Sum3/2
  Sum3/1 -> Mux/2  "f_bs"
  Trigonometric Function1/1 -> Product1/1
  Sum/1 -> Mux/1  "f_as"
  Trigonometric Function3/1 -> Product3/1
  Product3/1 -> Sum3/1
  Sum4/1 -> Trigonometric Function4/1
  Demux/1 -> Product2/2, Product3/2, Product/2  "f_qs^r"
  Demux/2 -> Product5/2, Product4/2, Product1/2  "f_ds^r"
  Demux/3 -> Sum/3, Sum6/3, Sum3/3  "f_0s"
  Sum1/1 -> Trigonometric Function3/1
  Sum5/1 -> Trigonometric Function5/1
  Trigonometric Function5/1 -> Product5/1
  Trigonometric Function2/1 -> Product2/1
  Product2/1 -> Sum6/1
  Product5/1 -> Sum6/2
  Sum2/1 -> Trigonometric Function2/1

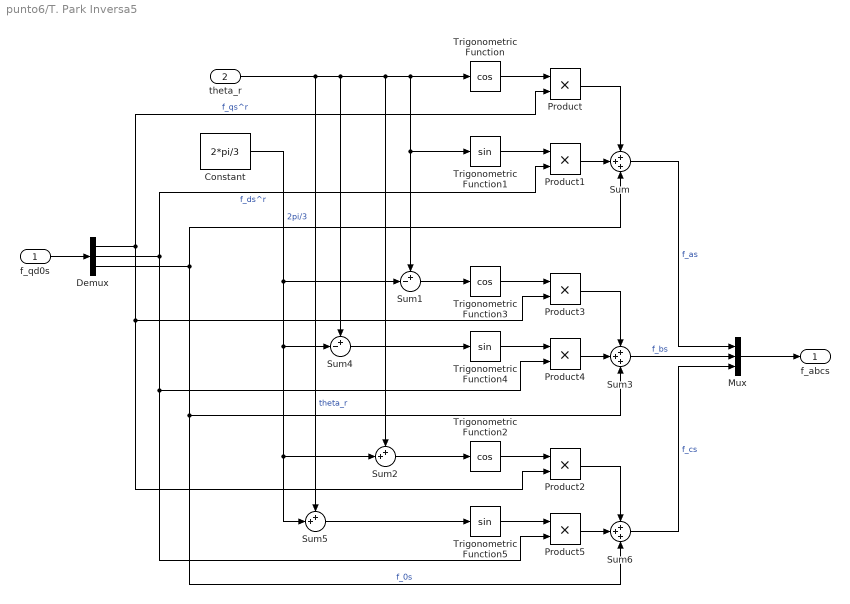
== system punto6/T. Park Inversa5 ==
  f_qd0s : Inport
  theta_r : Inport  Port=2
  Constant : Constant  Value=2*pi/3
  Demux : Demux  Outputs=3
  Mux : Mux  Inputs=3
  Product{,1..5} (6 alike) : Product
  Sum : Sum  Inputs=3
  Sum1 : Sum  Inputs=+-|
  Sum2 : Sum  Inputs=++|
  Sum3 : Sum  Inputs=3
  Sum4 : Sum  Inputs=+-|
  Sum5 : Sum  Inputs=++|
  Sum6 : Sum  Inputs=3
  Trigonometric Function : Trigonometry  Operator=cos
  Trigonometric Function1 : Trigonometry
  Trigonometric Function2 : Trigonometry  Operator=cos
  Trigonometric Function3 : Trigonometry  Operator=cos
  Trigonometric Function4 : Trigonometry
  Trigonometric Function5 : Trigonometry
  f_abcs : Outport  VectorParamsAs1DForOutWhenUnconnected=on
  wires:
  Trigonometric Function4/1 -> Product4/1
  f_qd0s/1 -> Demux/1
  Trigonometric Function/1 -> Product/1
  Constant/1 -> Sum1/2, Sum4/2, Sum2/2, Sum5/2  "2pi/3"
  Product1/1 -> Sum/2
  Mux/1 -> f_abcs/1
  Sum6/1 -> Mux/3  "f_cs"
  Product/1 -> Sum/1
  theta_r/1 -> Trigonometric Function/1, Trigonometric Function1/1, Sum1/1, Sum2/1, Sum4/1, Sum5/1  "theta_r"
  Product4/1 -> Sum3/2
  Sum3/1 -> Mux/2  "f_bs"
  Trigonometric Function1/1 -> Product1/1
  Sum/1 -> Mux/1  "f_as"
  Trigonometric Function3/1 -> Product3/1
  Product3/1 -> Sum3/1
  Sum4/1 -> Trigonometric Function4/1
  Demux/1 -> Product2/2, Product3/2, Product/2  "f_qs^r"
  Demux/2 -> Product5/2, Product4/2, Product1/2  "f_ds^r"
  Demux/3 -> Sum/3, Sum6/3, Sum3/3  "f_0s"
  Sum1/1 -> Trigonometric Function3/1
  Sum5/1 -> Trigonometric Function5/1
  Trigonometric Function5/1 -> Product5/1
  Trigonometric Function2/1 -> Product2/1
  Product2/1 -> Sum6/1
  Product5/1 -> Sum6/2
  Sum2/1 -> Trigonometric Function2/1

== system punto6/Ley control ids/Ley de Control minima ==
  Iqs : Inport
  wm : Inport  Port=2
  " 1" : Gain  Gain=Lq
  " 2" : Gain  Gain=Pp
  Product : Product
  Vds* : Outport
  wires:
  Iqs/1 -> " 1"/1  "iqs"
  " 1"/1 -> " 2"/1
  " 2"/1 -> Product/2
  wm/1 -> Product/1  "iqs"
  Product/1 -> Vds*/1

== system punto6/Ley control ids1/Ley de Control minima ==
  Iqs : Inport
  wm : Inport  Port=2
  " 1" : Gain  Gain=Lq
  " 2" : Gain  Gain=Pp
  Product : Product
  Vds* : Outport
  wires:
  Iqs/1 -> " 1"/1  "iqs"
  " 1"/1 -> " 2"/1
  " 2"/1 -> Product/2
  wm/1 -> Product/1  "iqs"
  Product/1 -> Vds*/1

== system punto6/SubsistemaTermico/Rs(t) ==
  Ts : Inport
  Rs_ref : Gain  Gain=1.02
  Sum5 : Sum  Inputs=|+-
  Sum6 : Sum  Inputs=|++
  Ts_ref : Constant  Value=40
  alfa_cu : Gain  Gain=alfa_cu
  cte : Constant
  Rs : Outport
  wires:
  alfa_cu/1 -> Sum6/1
  Sum6/1 -> Rs_ref/1
  Rs_ref/1 -> Rs/1  "Rs"
  Ts_ref/1 -> Sum5/2
  cte/1 -> Sum6/2
  Ts/1 -> Sum5/1
  Sum5/1 -> alfa_cu/1

== system punto6/SubsistemaTermico1/Rs(t) ==
  Ts : Inport
  Rs_ref : Gain  Gain=1.02
  Sum5 : Sum  Inputs=|+-
  Sum6 : Sum  Inputs=|++
  Ts_ref : Constant  Value=40
  alfa_cu : Gain  Gain=alfa_cu
  cte : Constant
  Rs : Outport
  wires:
  alfa_cu/1 -> Sum6/1
  Sum6/1 -> Rs_ref/1
  Rs_ref/1 -> Rs/1  "Rs"
  Ts_ref/1 -> Sum5/2
  cte/1 -> Sum6/2
  Ts/1 -> Sum5/1
  Sum5/1 -> alfa_cu/1
